simulink model "Damsim"  (R2019b)
settings: Solver=VariableStepAuto  StartTime=0.0  StopTime=sim_time  RelTol=1e-3
values from neighbouring files (symbols this model uses):
  A_mat_d = [0   1 ... (first row only)    [Dam_matlab_mscript.m]
  A_mat_m = [-D/J   Kt/J ... (first row only)    [Dam_matlab_mscript.m]
  A_mat_wl = [0]    [Dam_matlab_mscript.m]
  Ar = lr*wr    (= 10000)    [Dam_matlab_mscript.m]
  B_mat_d = [0  0 ... (first row only)    [Dam_matlab_mscript.m]
  B_mat_m = [0 ... (first row only)    [Dam_matlab_mscript.m]
  B_mat_wl = [Q]    [Dam_matlab_mscript.m]
  C_mat_d = [1 0]    [Dam_matlab_mscript.m]
  C_mat_m = [0  Kt]    [Dam_matlab_mscript.m]
  C_mat_wl = [1]    [Dam_matlab_mscript.m]
  D = 1.265    [Dam_matlab_mscript.m]
  D_mat_d = [0 0]    [Dam_matlab_mscript.m]
  D_mat_m = 0    [Dam_matlab_mscript.m]
  D_mat_wl = [0]    [Dam_matlab_mscript.m]
  g = 9.81    [Dam_matlab_mscript.m]
  J = 0.0005    [Dam_matlab_mscript.m]
  Kb = 0.33    [Dam_matlab_mscript.m]
  Kt = 2.47    [Dam_matlab_mscript.m]
  L = 0.00023    [Dam_matlab_mscript.m]
  lm = 2    [Dam_matlab_mscript.m]
  M = 3800    [Dam_matlab_mscript.m]
  N1 = 125    [Dam_matlab_mscript.m]
  N2 = 1250    [Dam_matlab_mscript.m]
  R = 0.025    [Dam_matlab_mscript.m]
  rp = 0.375    [Dam_matlab_mscript.m]
  slope = 4550    [Dam_matlab_mscript.m]
  Step_input = 400    [Dam_matlab_mscript.m]
  step_time = 0.1    [Dam_matlab_mscript.m]
  vw = 75    [Dam_matlab_mscript.m]
undefined symbols (not defined in the file or in its folder): den, den1, den2, den3, num, num1, num2, num3
libraries: simulink x1
settings Model: Creator=aravi  LastModifiedBy=aravi
settings DataIOCC: ReturnWorkspaceOutputs=off

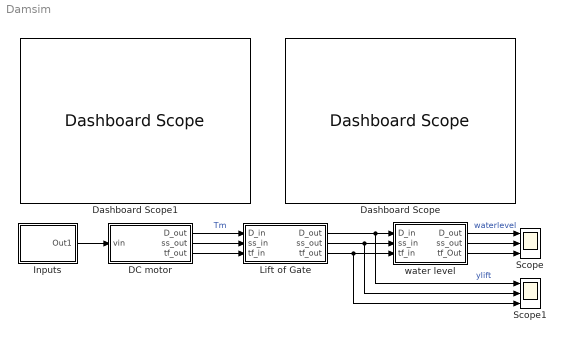
== system Damsim ==
  DC motor : Subsystem
  Dashboard Scope : DashboardScope  Ymax=21
  Dashboard Scope1 : DashboardScope
  Inputs : Subsystem
  Lift of Gate : Subsystem
  Scope : Scope  NumInputPorts=3
  Scope1 : Scope  NumInputPorts=3
  water level : Subsystem
  wires:
  water level/1(D_out) -> Scope/1  "waterlevel"
  water level/3(tf_Out) -> Scope/3
  water level/2(ss_out) -> Scope/2
  Lift of Gate/1(D_out) -> Scope1/1, water level/1(D_in)  "ylift"
  DC motor/1(D_out) -> Lift of Gate/1(D_in)  "Tm"
  DC motor/2(ss_out) -> Lift of Gate/2(ss_in)
  DC motor/3(tf_out) -> Lift of Gate/3(tf_in)
  Lift of Gate/3(tf_out) -> water level/3(tf_in), Scope1/3
  Lift of Gate/2(ss_out) -> Scope1/2, water level/2(ss_in)
  Inputs/1(Out1) -> DC motor/1(vin)

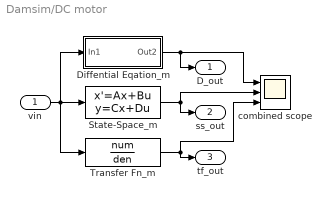
== system Damsim/DC motor ==
  vin : Inport
  Diffential Eqation_m : Subsystem
  "State-Space_m " : StateSpace  A=A_mat_m  B=B_mat_m  C=C_mat_m  D=D_mat_m  InitialCondition=0
  Transfer Fn_m : TransferFcn  Numerator=num  Denominator=den
  combined scope : Scope  NumInputPorts=3
  D_out : Outport
  ss_out : Outport  Port=2
  tf_out : Outport  Port=3
  wires:
  Transfer Fn_m/1 -> tf_out/1, combined scope/3
  "State-Space_m "/1 -> combined scope/2, ss_out/1
  vin/1 -> Diffential Eqation_m/1(In1), Transfer Fn_m/1, "State-Space_m "/1
  Diffential Eqation_m/1(Out2) -> combined scope/1, D_out/1

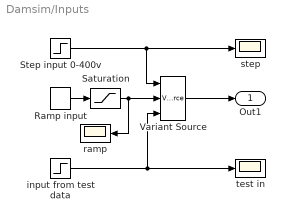
== system Damsim/Inputs ==
  " input from test data" : Step  Time=0  After=400  SampleTime=0
  "Ramp input " : simulink/Sources/Ramp  slope=slope  start=0.1  InitialOutput=0
  Saturation : Saturate  UpperLimit=400  LowerLimit=0
  Step input 0-400v : Step  Time=step_time  After=Step_input  SampleTime=0
  "Variant Source " : VariantSource
  ramp : Scope
  step : Scope
  test in : Scope
  Out1 : Outport
  wires:
  "Ramp input "/1 -> Saturation/1
  Step input 0-400v/1 -> "Variant Source "/1, step/1
  Saturation/1 -> ramp/1, "Variant Source "/2
  "Variant Source "/1 -> Out1/1
  " input from test data"/1 -> test in/1, "Variant Source "/3

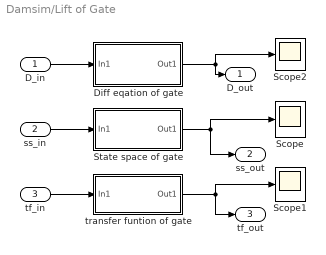
== system Damsim/Lift of Gate ==
  D_in : Inport
  ss_in : Inport  Port=2
  tf_in : Inport  Port=3
  Diff eqation of gate : Subsystem
  Scope : Scope
  Scope1 : Scope
  Scope2 : Scope
  State space of gate : Subsystem
  transfer funtion of gate : Subsystem
  D_out : Outport
  ss_out : Outport  Port=2
  tf_out : Outport  Port=3
  wires:
  transfer funtion of gate/1(Out1) -> tf_out/1, Scope1/1
  State space of gate/1(Out1) -> ss_out/1, Scope/1
  Diff eqation of gate/1(Out1) -> D_out/1, Scope2/1
  D_in/1 -> Diff eqation of gate/1(In1)
  ss_in/1 -> State space of gate/1(In1)
  tf_in/1 -> transfer funtion of gate/1(In1)

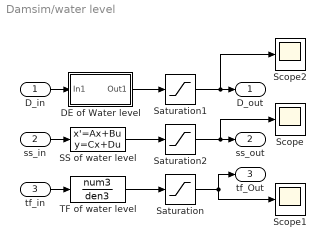
== system Damsim/water level ==
  D_in : Inport
  ss_in : Inport  Port=2
  tf_in : Inport  Port=3
  DE of Water level : Subsystem
  SS of water level : StateSpace  A=A_mat_wl  B=B_mat_wl  C=C_mat_wl  D=D_mat_wl  InitialCondition=0
  Saturation : Saturate  UpperLimit=20  LowerLimit=0
  Saturation1 : Saturate  UpperLimit=20
  Saturation2 : Saturate  UpperLimit=20  LowerLimit=0
  Scope : Scope
  Scope1 : Scope
  Scope2 : Scope
  TF of water level : TransferFcn  Numerator=num3  Denominator=den3
  D_out : Outport
  ss_out : Outport  Port=2
  tf_Out : Outport  Port=3
  wires:
  D_in/1 -> DE of Water level/1(In1)
  ss_in/1 -> SS of water level/1
  SS of water level/1 -> Saturation2/1
  Saturation/1 -> Scope1/1, tf_Out/1
  TF of water level/1 -> Saturation/1
  tf_in/1 -> TF of water level/1
  DE of Water level/1(Out1) -> Saturation1/1
  Saturation1/1 -> Scope2/1, D_out/1
  Saturation2/1 -> Scope/1, ss_out/1

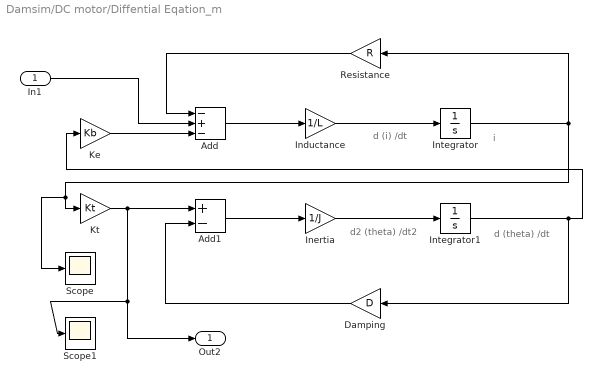
== system Damsim/DC motor/Diffential Eqation_m ==
  note: i
  note: d2 (theta) /dt2
  note: d (i) /dt
  note: d (theta) /dt
  In1 : Inport
  Add : Sum  Inputs=-+-
  Add1 : Sum  Inputs=+-
  Damping : Gain  Gain=D
  Inductance : Gain  Gain=1/L
  Inertia : Gain  Gain=1/J
  Integrator : Integrator
  Integrator1 : Integrator
  Ke : Gain  Gain=Kb
  Kt : Gain  Gain=Kt
  Resistance : Gain  Gain=R
  Scope : Scope
  Scope1 : Scope
  Out2 : Outport
  wires:
  Ke/1 -> Add/3
  Resistance/1 -> Add/1
  Kt/1 -> Scope1/1, Out2/1, Add1/1
  Integrator1/1 -> Damping/1, Ke/1
  Integrator/1 -> Resistance/1, Scope/1, Kt/1
  Add1/1 -> Inertia/1
  Inertia/1 -> Integrator1/1
  Add/1 -> Inductance/1
  Inductance/1 -> Integrator/1
  Damping/1 -> Add1/2
  In1/1 -> Add/2

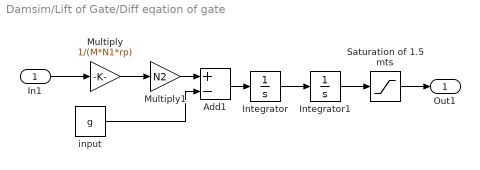
== system Damsim/Lift of Gate/Diff eqation of gate ==
  In1 : Inport
  Add1 : Sum  Inputs=+-
  Integrator : Integrator
  Integrator1 : Integrator
  Multiply : Gain  Gain=1/(M*N1*rp)
  Multiply1 : Gain  Gain=N2
  Saturation of 1.5 mts : Saturate  UpperLimit=1.5  LowerLimit=0
  input : Constant  Value=g
  Out1 : Outport
  wires:
  In1/1 -> Multiply/1
  input/1 -> Add1/2
  Integrator1/1 -> Saturation of 1.5 mts/1
  Add1/1 -> Integrator/1
  Saturation of 1.5 mts/1 -> Out1/1
  Multiply/1 -> Multiply1/1
  Multiply1/1 -> Add1/1
  Integrator/1 -> Integrator1/1

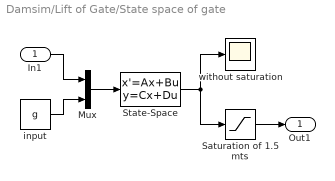
== system Damsim/Lift of Gate/State space of gate ==
  In1 : Inport
  Mux : Mux  Inputs=2
      settings: DisplayOption=signals
  Saturation of 1.5 mts : Saturate  UpperLimit=1.5  LowerLimit=0
  State-Space : StateSpace  A=A_mat_d  B=B_mat_d  C=C_mat_d  D=D_mat_d  InitialCondition=0
  input : Constant  Value=g
  without saturation : Scope
  Out1 : Outport
  wires:
  Mux/1 -> State-Space/1
  input/1 -> Mux/2
  In1/1 -> Mux/1
  State-Space/1 -> Saturation of 1.5 mts/1, without saturation/1
  Saturation of 1.5 mts/1 -> Out1/1

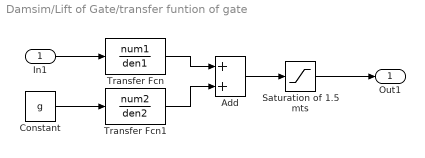
== system Damsim/Lift of Gate/transfer funtion of gate ==
  In1 : Inport
  Add : Sum
  Constant : Constant  Value=g
  Saturation of 1.5 mts : Saturate  UpperLimit=1.5  LowerLimit=0
  Transfer Fcn : TransferFcn  Numerator=num1  Denominator=den1
  Transfer Fcn1 : TransferFcn  Numerator=num2  Denominator=den2
  Out1 : Outport
  wires:
  Constant/1 -> Transfer Fcn1/1
  Transfer Fcn/1 -> Add/1
  Transfer Fcn1/1 -> Add/2
  Add/1 -> Saturation of 1.5 mts/1
  In1/1 -> Transfer Fcn/1
  Saturation of 1.5 mts/1 -> Out1/1

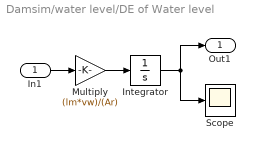
== system Damsim/water level/DE of Water level ==
  In1 : Inport
  Integrator : Integrator
  Multiply : Gain  Gain=(lm*vw)/(Ar)
  Scope : Scope
  Out1 : Outport
  wires:
  Multiply/1 -> Integrator/1
  In1/1 -> Multiply/1
  Integrator/1 -> Out1/1, Scope/1
